simulink model "sys_fcn"  (R2020b)
settings: Solver=VariableStepAuto  StartTime=0.0  StopTime=50  RelTol=1e-3
libraries: simulink x2
settings Model: Creator=zhiyao  LastModifiedBy=zhiyao

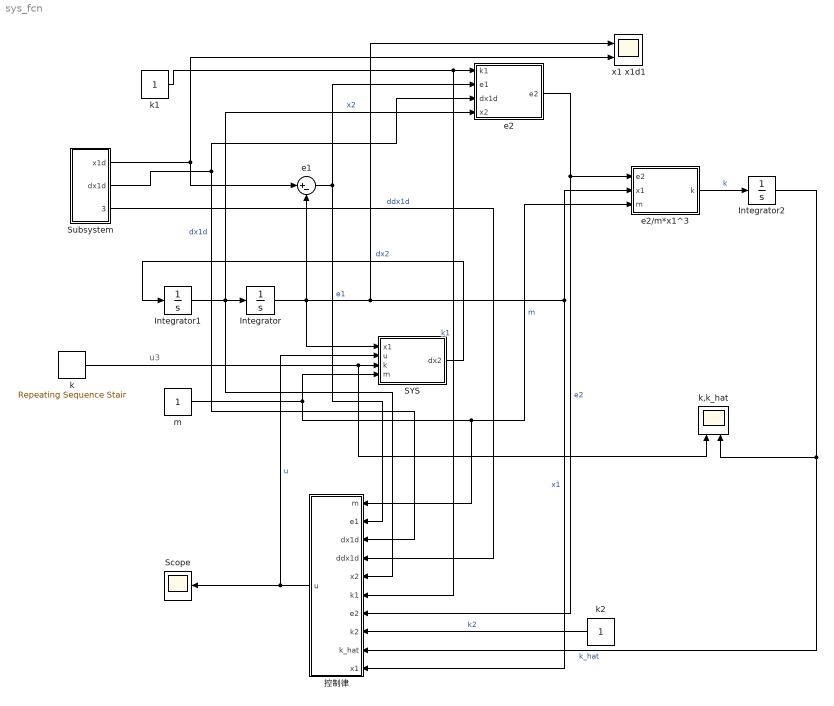
== system sys_fcn ==
  note: u3
  Integrator : Integrator
  Integrator1 : Integrator
  Integrator2 : Integrator
  SYS : MATLAB Function  TreatAsAtomicUnit=on
  Scope : Scope
  Subsystem : Subsystem
  e1 : Sum  Inputs=|+-
  e2 : MATLAB Function  TreatAsAtomicUnit=on
  e2/m*x1^3 : MATLAB Function  TreatAsAtomicUnit=on
  k : simulink/Sources/Repeating Sequence Stair  OutValues=[8].'  tsamp=25  OutMin=[]  OutMax=[]  OutDataTypeStr=double  OutputDataTypeScalingMode=double  OutDataType=fixdt(0,8)  ConRadixGroup=Best Precision: Vector-wise  OutScaling=2^-12
  k,k_hat : Scope  NumInputPorts=2
  k1 : Constant
  k2 : Constant
  m : Constant
  x1 x1d1 : Scope  NumInputPorts=2
  控制律 : MATLAB Function  TreatAsAtomicUnit=on
  wires:
  m/1 -> SYS/4(m), 控制律/1(m), e2/m*x1^3/3(m)  "m"
  Integrator/1 -> SYS/1(x1), x1 x1d1/1, 控制律/10(x1), e2/m*x1^3/2(x1), e1/2  "x1"
  控制律/1(u) -> Scope/1, SYS/2(u)  "u"
  Integrator1/1 -> 控制律/5(x2), e2/4(x2), Integrator/1  "x2"
  Subsystem/1(x1d) -> e1/1, x1 x1d1/2
  e1/1 -> 控制律/2(e1), e2/2(e1)  "e1"
  k1/1 -> 控制律/6(k1), e2/1(k1)  "k1"
  Subsystem/2(dx1d) -> 控制律/3(dx1d), e2/3(dx1d)  "dx1d"
  SYS/1(dx2) -> Integrator1/1  "dx2"
  e2/m*x1^3/1(k) -> Integrator2/1  "k"
  Integrator2/1 -> 控制律/9(k_hat), k,k_hat/2  "k_hat"
  e2/1(e2) -> 控制律/7(e2), e2/m*x1^3/1(e2)  "e2"
  Subsystem/3(ddx1d) -> 控制律/4(ddx1d)  "ddx1d"
  k2/1 -> 控制律/8(k2)  "k2"
  k/1 -> k,k_hat/1, SYS/3(k)

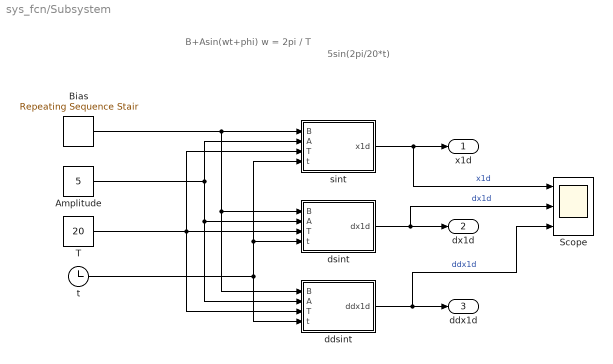
== system sys_fcn/Subsystem ==
  note: 5sin(2pi/20*t)
  note: B+Asin(wt+phi)
      | w = 2pi / T
  Amplitude : Constant  Value=5
  Bias : simulink/Sources/Repeating Sequence Stair  OutValues=[0,1,2,3,4].'  tsamp=10  OutMin=[]  OutMax=[]  OutDataTypeStr=double  OutputDataTypeScalingMode=double  OutDataType=fixdt(0,8)  ConRadixGroup=Best Precision: Vector-wise  OutScaling=2^-12
  Scope : Scope  NumInputPorts=3
  T : Constant  Value=20
  ddsint : MATLAB Function  TreatAsAtomicUnit=on
  dsint : MATLAB Function  TreatAsAtomicUnit=on
  sint : MATLAB Function  TreatAsAtomicUnit=on
  t : Clock
  x1d : Outport
  dx1d : Outport  Port=2
  ddx1d : Outport  Port=3
  wires:
  Bias/1 -> ddsint/1(B), dsint/1(B), sint/1(B)
  t/1 -> ddsint/4(t), dsint/4(t), sint/4(t)
  Amplitude/1 -> ddsint/2(A), dsint/2(A), sint/2(A)
  T/1 -> sint/3(T), ddsint/3(T), dsint/3(T)
  sint/1(x1d) -> Scope/1, x1d/1  "x1d"
  ddsint/1(ddx1d) -> Scope/3, ddx1d/1  "ddx1d"
  dsint/1(dx1d) -> Scope/2, dx1d/1  "dx1d"

== matlab function sys_fcn/控制律 ==
  data: m input; u output; e1 input; dx1d input; ddx1d input; x2 input; k1 input; e2 input; k2 input; k_hat input; x1 input
function u = fcn(m,e1,dx1d,ddx1d,x2,k1,e2,k2,k_hat,x1)

u = m*e1+m*ddx1d+m*k1*(dx1d-x2)+k_hat*x1^3+m*k2*e2;

== matlab function sys_fcn/SYS ==
  data: x1 input; u input; dx2 output; k input; m input
function dx2 = fcn(x1,u,k,m)

dx2 =-k/m*(x1)^3+1/m*u;

== matlab function sys_fcn/e2 ==
  data: e2 output; k1 input; e1 input; dx1d input; x2 input
function e2 = fc(k1,e1,dx1d,x2)

e2 = dx1d+k1*e1-x2;

== matlab function sys_fcn/e2//m*x1^3 ==
  data: e2 input; k output; x1 input; m input
function k = fcn(e2,x1,m)

k = e2/m*(x1)^3;

== matlab function sys_fcn/Subsystem/sint ==
  data: B input; x1d output; A input; T input; t input
function x1d = fc(B,A,T,t)

x1d = B+A*sin(2*pi/T*t);

== matlab function sys_fcn/Subsystem/dsint ==
  data: B input; dx1d output; A input; T input; t input
function dx1d = fc(B,A,T,t)

dx1d = A*2*pi/T*cos(2*pi/T*t);

== matlab function sys_fcn/Subsystem/ddsint ==
  data: B input; ddx1d output; A input; T input; t input
function ddx1d = fc(B,A,T,t)

ddx1d = -2*pi/T*A*2*pi/T*sin(2*pi/T*t);
